simulink model "time_test"  (R2018b)
settings: Solver=VariableStepAuto  StartTime=0.0  StopTime=0  FixedStep=.2  RelTol=1e-3
values from neighbouring files (symbols this model uses):
  j_seconds = (JDutc_in - fswParams.constants.global.JDJ2000)*fswParams.constants.convert.DAY2SEC    [time_test_init.m]
libraries: time_Lib x1
settings Model: Creator=devantormey  LastModifiedBy=devantormey

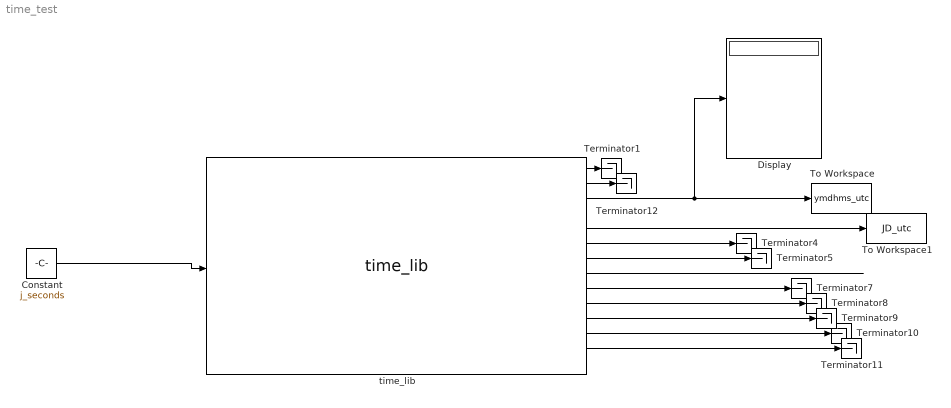
== system time_test ==
  Constant : Constant  Value=j_seconds
  Display : Display
  Terminator{1,4..5,7..12} (9 alike) : Terminator
  To Workspace : ToWorkspace  VariableName=ymdhms_utc  SaveFormat=Timeseries  SampleTime=-1
  To Workspace1 : ToWorkspace  VariableName=JD_utc  SaveFormat=Timeseries  SampleTime=-1
  "time_lib " : time_Lib/time_lib    SystemSampleTime=-1
  wires:
  Constant/1 -> "time_lib "/1
  "time_lib "/2 -> Terminator12/1
  "time_lib "/3 -> Display/1, To Workspace/1
  "time_lib "/6 -> Terminator4/1
  "time_lib "/7 -> Terminator5/1
  "time_lib "/8 -> ?
  "time_lib "/9 -> Terminator7/1
  "time_lib "/10 -> Terminator8/1
  "time_lib "/11 -> Terminator9/1
  "time_lib "/12 -> Terminator10/1
  "time_lib "/13 -> Terminator11/1
  "time_lib "/1 -> Terminator1/1
  "time_lib "/5 -> To Workspace1/1
